simulink model "FLC_sim_tune_Ke"  (R2023a)
settings: Solver=VariableStepAuto  StartTime=0.0  StopTime=10.0  RelTol=1e-3
libraries: fuzblock x4
settings Model: Creator=dimal  LastModifiedBy=dimal

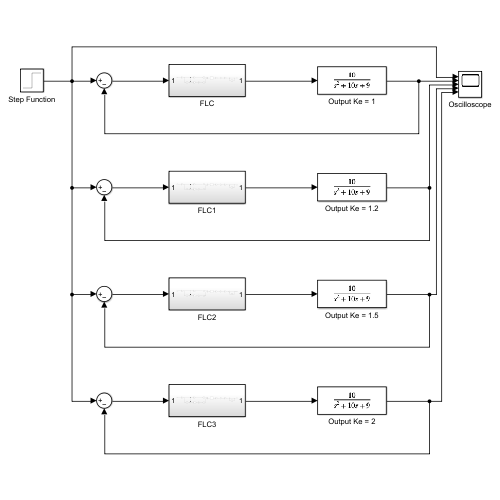
[thumbnail: Simulink's stored preview of the top-level diagram]
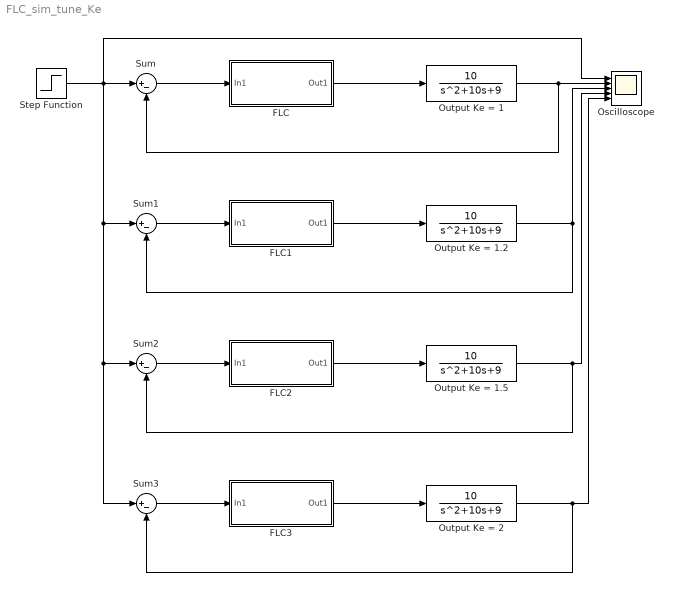
== system FLC_sim_tune_Ke ==
  FLC : Subsystem
  FLC1 : Subsystem
  FLC2 : Subsystem
  FLC3 : Subsystem
  Oscilloscope : Scope  NumInputPorts=5
  Output Ke = 1 : TransferFcn  Numerator=[10]  Denominator=[1 10 9]
  Output Ke = 1.2 : TransferFcn  Numerator=[10]  Denominator=[1 10 9]
  Output Ke = 1.5 : TransferFcn  Numerator=[10]  Denominator=[1 10 9]
  Output Ke = 2 : TransferFcn  Numerator=[10]  Denominator=[1 10 9]
  Step Function : Step  Time=0  After=60  SampleTime=0.01
  Sum{,1..3} (4 alike) : Sum  Inputs=|+-
  wires:
  FLC/1(Out1) -> Output Ke = 1/1
  Sum/1 -> FLC/1(In1)
  Step Function/1 -> Sum1/1, Sum3/1, Sum2/1, Oscilloscope/1, Sum/1
  Output Ke = 1/1 -> Oscilloscope/2, Sum/2
  FLC1/1(Out1) -> Output Ke = 1.2/1
  Output Ke = 1.2/1 -> Sum1/2, Oscilloscope/3
  Sum1/1 -> FLC1/1(In1)
  Output Ke = 1.5/1 -> Oscilloscope/4, Sum2/2
  FLC2/1(Out1) -> Output Ke = 1.5/1
  Sum2/1 -> FLC2/1(In1)
  Output Ke = 2/1 -> Oscilloscope/5, Sum3/2
  FLC3/1(Out1) -> Output Ke = 2/1
  Sum3/1 -> FLC3/1(In1)

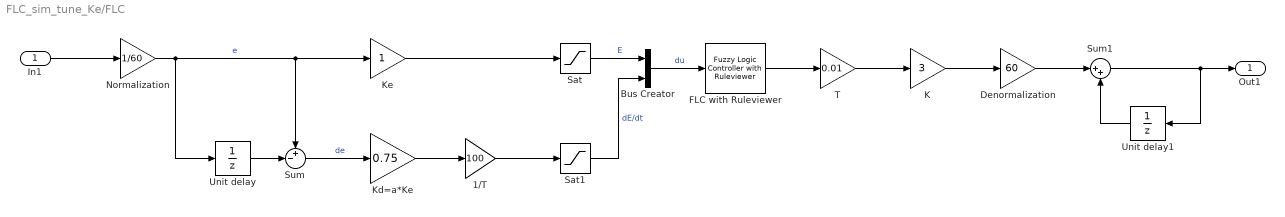
== system FLC_sim_tune_Ke/FLC ==
  In1 : Inport
  1/T : Gain  Gain=100
  Bus Creator : BusCreator  Inputs=2
  Denormalization : Gain  Gain=60
  FLC with Ruleviewer : fuzblock/Fuzzy Logic  Controller  with Ruleviewer  fismatrix=FLC  Ts=2
  K : Gain  Gain=3
  Kd=a*Ke : Gain  Gain=0.75
  Ke : Gain
  Normalization : Gain  Gain=1/60
  Sat : Saturate
  Sat1 : Saturate
  Sum : Sum  Inputs=+-|
  Sum1 : Sum  Inputs=|++
  T : Gain  Gain=0.01
  Unit delay : UnitDelay  SampleTime=-1  HasFrameUpgradeWarning=on
  Unit delay1 : UnitDelay  SampleTime=-1  HasFrameUpgradeWarning=on
  Out1 : Outport
  wires:
  Normalization/1 -> Unit delay/1, Sum/1, Ke/1  "e"
  Ke/1 -> Sat/1
  Sum/1 -> Kd=a*Ke/1  "de"
  Kd=a*Ke/1 -> 1/T/1
  1/T/1 -> Sat1/1
  Sat/1 -> Bus Creator/1  "E"
  Sat1/1 -> Bus Creator/2  "dE/dt"
  FLC with Ruleviewer/1 -> T/1
  T/1 -> K/1
  K/1 -> Denormalization/1
  Denormalization/1 -> Sum1/1
  Unit delay/1 -> Sum/2
  Sum1/1 -> Out1/1, Unit delay1/1
  Unit delay1/1 -> Sum1/2
  In1/1 -> Normalization/1
  Bus Creator/1 -> FLC with Ruleviewer/1  "du"

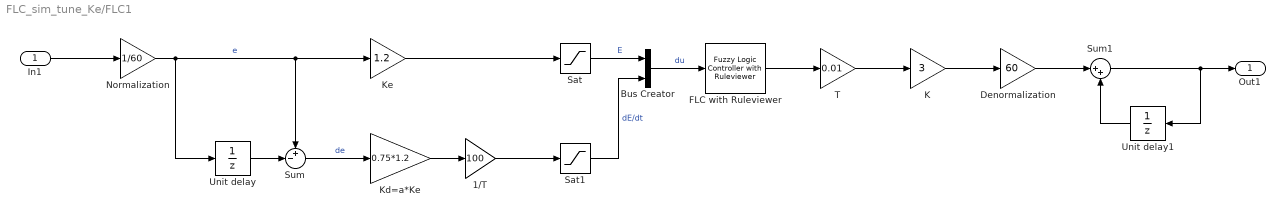
== system FLC_sim_tune_Ke/FLC1 ==
  In1 : Inport
  1/T : Gain  Gain=100
  Bus Creator : BusCreator  Inputs=2
  Denormalization : Gain  Gain=60
  FLC with Ruleviewer : fuzblock/Fuzzy Logic  Controller  with Ruleviewer  fismatrix=FLC  Ts=2
  K : Gain  Gain=3
  Kd=a*Ke : Gain  Gain=0.75*1.2
  Ke : Gain  Gain=1.2
  Normalization : Gain  Gain=1/60
  Sat : Saturate
  Sat1 : Saturate
  Sum : Sum  Inputs=+-|
  Sum1 : Sum  Inputs=|++
  T : Gain  Gain=0.01
  Unit delay : UnitDelay  SampleTime=-1  HasFrameUpgradeWarning=on
  Unit delay1 : UnitDelay  SampleTime=-1  HasFrameUpgradeWarning=on
  Out1 : Outport
  wires:
  Normalization/1 -> Unit delay/1, Sum/1, Ke/1  "e"
  Ke/1 -> Sat/1
  Sum/1 -> Kd=a*Ke/1  "de"
  Kd=a*Ke/1 -> 1/T/1
  1/T/1 -> Sat1/1
  Sat/1 -> Bus Creator/1  "E"
  Sat1/1 -> Bus Creator/2  "dE/dt"
  FLC with Ruleviewer/1 -> T/1
  T/1 -> K/1
  K/1 -> Denormalization/1
  Denormalization/1 -> Sum1/1
  Unit delay/1 -> Sum/2
  Sum1/1 -> Out1/1, Unit delay1/1
  Unit delay1/1 -> Sum1/2
  In1/1 -> Normalization/1
  Bus Creator/1 -> FLC with Ruleviewer/1  "du"

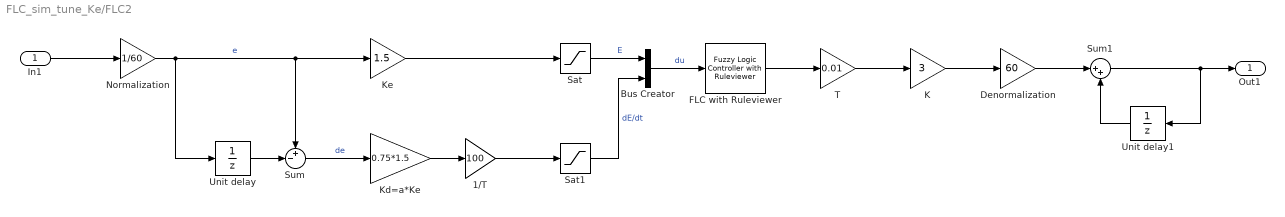
== system FLC_sim_tune_Ke/FLC2 ==
  In1 : Inport
  1/T : Gain  Gain=100
  Bus Creator : BusCreator  Inputs=2
  Denormalization : Gain  Gain=60
  FLC with Ruleviewer : fuzblock/Fuzzy Logic  Controller  with Ruleviewer  fismatrix=FLC  Ts=2
  K : Gain  Gain=3
  Kd=a*Ke : Gain  Gain=0.75*1.5
  Ke : Gain  Gain=1.5
  Normalization : Gain  Gain=1/60
  Sat : Saturate
  Sat1 : Saturate
  Sum : Sum  Inputs=+-|
  Sum1 : Sum  Inputs=|++
  T : Gain  Gain=0.01
  Unit delay : UnitDelay  SampleTime=-1  HasFrameUpgradeWarning=on
  Unit delay1 : UnitDelay  SampleTime=-1  HasFrameUpgradeWarning=on
  Out1 : Outport
  wires:
  Normalization/1 -> Unit delay/1, Sum/1, Ke/1  "e"
  Ke/1 -> Sat/1
  Sum/1 -> Kd=a*Ke/1  "de"
  Kd=a*Ke/1 -> 1/T/1
  1/T/1 -> Sat1/1
  Sat/1 -> Bus Creator/1  "E"
  Sat1/1 -> Bus Creator/2  "dE/dt"
  FLC with Ruleviewer/1 -> T/1
  T/1 -> K/1
  K/1 -> Denormalization/1
  Denormalization/1 -> Sum1/1
  Unit delay/1 -> Sum/2
  Sum1/1 -> Out1/1, Unit delay1/1
  Unit delay1/1 -> Sum1/2
  In1/1 -> Normalization/1
  Bus Creator/1 -> FLC with Ruleviewer/1  "du"

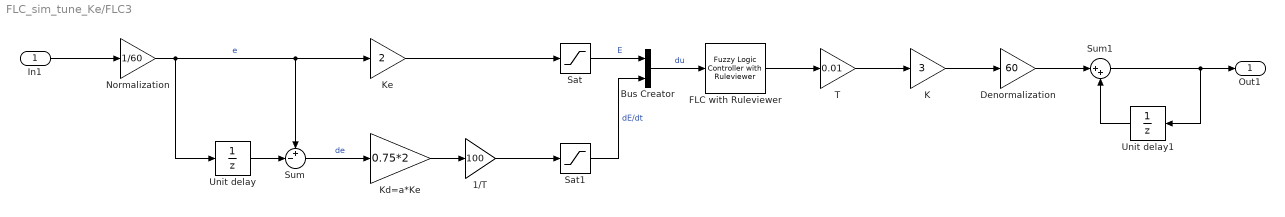
== system FLC_sim_tune_Ke/FLC3 ==
  In1 : Inport
  1/T : Gain  Gain=100
  Bus Creator : BusCreator  Inputs=2
  Denormalization : Gain  Gain=60
  FLC with Ruleviewer : fuzblock/Fuzzy Logic  Controller  with Ruleviewer  fismatrix=FLC  Ts=2
  K : Gain  Gain=3
  Kd=a*Ke : Gain  Gain=0.75*2
  Ke : Gain  Gain=2
  Normalization : Gain  Gain=1/60
  Sat : Saturate
  Sat1 : Saturate
  Sum : Sum  Inputs=+-|
  Sum1 : Sum  Inputs=|++
  T : Gain  Gain=0.01
  Unit delay : UnitDelay  SampleTime=-1  HasFrameUpgradeWarning=on
  Unit delay1 : UnitDelay  SampleTime=-1  HasFrameUpgradeWarning=on
  Out1 : Outport
  wires:
  Normalization/1 -> Unit delay/1, Sum/1, Ke/1  "e"
  Ke/1 -> Sat/1
  Sum/1 -> Kd=a*Ke/1  "de"
  Kd=a*Ke/1 -> 1/T/1
  1/T/1 -> Sat1/1
  Sat/1 -> Bus Creator/1  "E"
  Sat1/1 -> Bus Creator/2  "dE/dt"
  FLC with Ruleviewer/1 -> T/1
  T/1 -> K/1
  K/1 -> Denormalization/1
  Denormalization/1 -> Sum1/1
  Unit delay/1 -> Sum/2
  Sum1/1 -> Out1/1, Unit delay1/1
  Unit delay1/1 -> Sum1/2
  In1/1 -> Normalization/1
  Bus Creator/1 -> FLC with Ruleviewer/1  "du"
